simulink subsystem "Radar"  (R2024b)
settings: Solver=VariableStepAuto  StartTime=0.0  StopTime=10.0  RelTol=1e-3
undefined symbols (not defined in the file or in its folder): rel_dist, rel_vel
libraries: drivinglib x1, sim3dcameralib x1, sim3dprobsensorlib x1
settings Model: Creator=Tong  LastModifiedBy=Tong

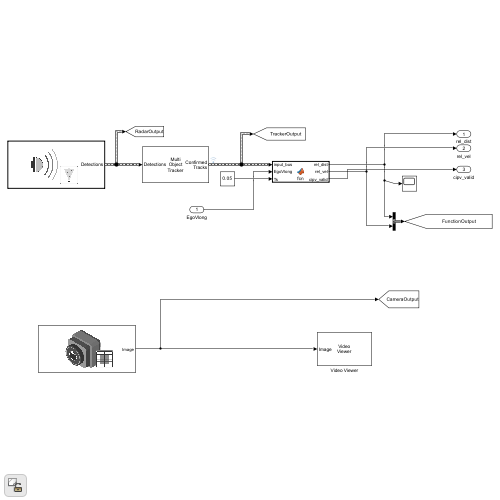
[thumbnail: Simulink's stored preview of the top-level diagram]
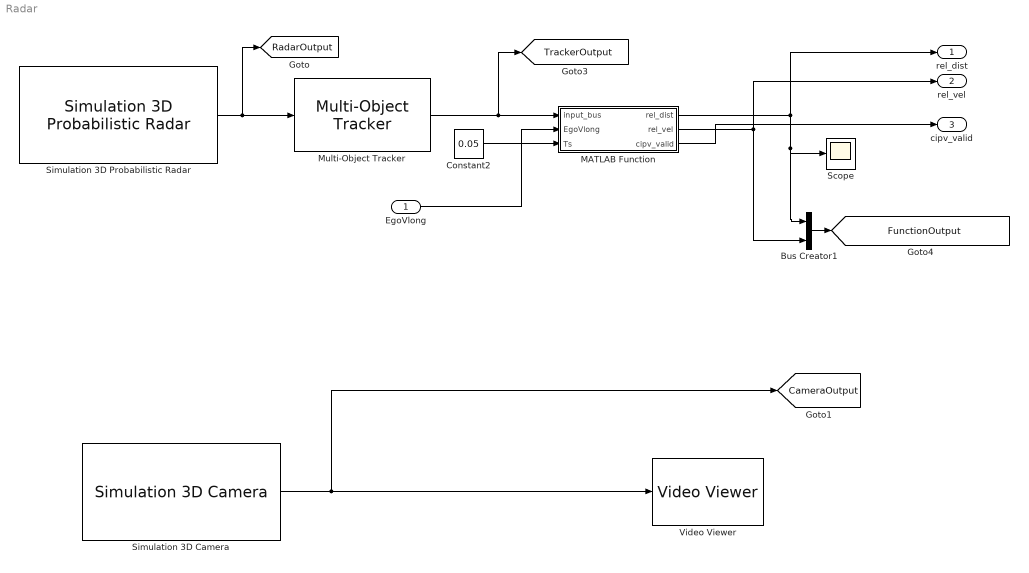
== system Radar ==
  EgoVlong : Inport
  Bus Creator1 : BusCreator  Inputs=rel_dist,rel_vel
  Constant2 : Constant  Value=0.05
  MATLAB Function : MATLAB Function  TreatAsAtomicUnit=on
  Multi-Object Tracker : drivinglib/Multi-Object Tracker  TrackerIndex=uint32( 0 )  FilterInitializationFcn=initcvekf  AssignmentThreshold=40  ConfirmationThreshold=[ 2, 3 ]  DeletionThreshold=[ 4, 5 ]  MaxNumTracks=50  MaxNumSensors=1  OOSMHandling=Terminate  StateParametersSimulink=struct  HasStateParametersInput=off  TimeInputSource=Auto  HasCostMatrixInput=off  HasDetectableTrackIDsInput=off  BusNameSource=Auto  BusName=BusMultiObjectTracker  TentativeTracksOutputPort=off  AllTracksOutputPort=off  SimulateUsing=Interpreted execution
  Scope : Scope
  Simulation 3D Camera : sim3dcameralib/Simulation 3D Camera  Priority=1  sensorTag=Sim3dSensor  sensorId=1  sensorName=Sim3dSensor  vehTagList={'Scene Origin'}  vehTag=Scene Origin  mountLoc=Hood center  offsetFlag=on  tmountOffset=[0, 0, 0]  extTmount=off  rmountOffset=[0, 0, 0]  extRmount=off  FocalLength=[1109, 1109]  OpticalCenter=[640, 360]  ImageSize=[720, 1280]  RadialDistortion=[0, 0]  TangentialDistortion=[0, 0]  SensorSkew=0  DepthOutportEnabled=off  SemanticOutportEnabled=off  TransformOutportEnabled=off  SampleTime=-1  mountPoint=[2.4735 0 0.44]  mountOrientation=[0 0 0]  aMode=3  ID=1
      settings: LibrarySourceBlock=drivingsim3d/Simulation 3D Camera
  Simulation 3D Probabilistic Radar : sim3dprobsensorlib/Simulation 3D Probabilistic Radar  Priority=1  sensorTag=Sim3dSensor  sensorId=2  sensorName=Sim3dSensor  vehTagList={'Scene Origin'}  vehTag=Scene Origin  mountLoc=Front bumper  offsetFlag=on  tmountOffset=[0.5, 0, 0.6]  rmountOffset=[0, 2, 0]  AzimuthResolution=4  ElevationResolution=5  RangeResolution=2.5  RangeRateResolution=0.5  AzimuthBiasFraction=0.1  ElevationBiasFraction=0.1  RangeBiasFraction=0.05  RangeRateBiasFraction=0.05  FieldOfView=[ 20, 6 ]  DetectionRange=[ 0.5, 150 ]  RangeRateLimits=[ -100, 100 ]  DetectionProbability=0.95  FalseAlarmRate=1e-7  ReferenceRange=200  ReferenceRCS=-15  HasElevation=on  HasRangeRate=on  HasNoise=off  HasFalseAlarms=off  InitialSeedSource=Repeatable  InitialSeed=0  MaxNumDetections=50  DetectionCoordinates=Ego Cartesian  SpecifyOutputBusName=off  BusName=BusSimulation3DRadarTruthSensor  SampleTime=0.05  mountPoint=[2.9735 0 1.04]  mountOrientation=[0 -2 0]  aMode=3  ID=2
      settings: LibrarySourceBlock=drivingsim3d/Simulation 3D Probabilistic Radar
  Video Viewer : VideoViewer  FigPos=[-8.33333333333333 995.333333333333 850.666666666667 403.333333333333]
  rel_dist : Outport
  rel_vel : Outport  Port=2
  cipv_valid : Outport  Port=3
  tag scope: CameraOutput=global, FunctionOutput=global, RadarOutput=global, TrackerOutput=global
  wires:
  Constant2/1 -> MATLAB Function/3(Ts)
  Bus Creator1/1 -> [FunctionOutput]
  Simulation 3D Probabilistic Radar/1 -> [RadarOutput], Multi-Object Tracker/1
  EgoVlong/1 -> MATLAB Function/2(EgoVlong)
  Multi-Object Tracker/1 -> MATLAB Function/1(input_bus), [TrackerOutput]
  MATLAB Function/2(rel_vel) -> rel_vel/1, Bus Creator1/2
  MATLAB Function/1(rel_dist) -> Bus Creator1/1, Scope/1, rel_dist/1
  MATLAB Function/3(cipv_valid) -> cipv_valid/1
  Simulation 3D Camera/1 -> Video Viewer/1, [CameraOutput]

== matlab function Radar/MATLAB Function ==
  settings: updateMethod=DISCRETE
  data: input_bus input; rel_dist output; rel_vel output; EgoVlong input; cipv_valid output; Ts input
function [rel_dist, rel_vel, cipv_valid] = fcn(input_bus, EgoVlong, Ts)
%#codegen
coder.extrinsic('fprintf');

% ===== 参数（按需调）=====
dNoTarget = 200;          % 无目标输出距离
dMaxOut   = 150;          % 认为有效输出的最大距离
max_coast_time = 0.5;     % 允许丢目标后靠预测维持的时间(s)
max_coast = int32(round(max_coast_time / Ts));

% KF 过程噪声（匀加速模型）
sigma_a = 2.0;            % m/s^2
% =========================

% ======= 持久变量 =======
persistent X_est P frame_count lost_count last_cipv_id inited
if isempty(inited)
    frame_count  = 0;
    lost_count   = int32(max_coast+1);  % 一开始当作无目标
    last_cipv_id = uint32(0);
    X_est = [dNoTarget; 0];
    P     = [100 0; 0 100];
    inited = true;
end

frame_count = frame_count + 1;

num_tracks  = double(input_bus.NumTracks);
tracks      = input_bus.Tracks;

% ======= 1) KF 预测 =======
dt = Ts;
A = [1 dt; 0 1];
Q = [0.25*dt^4  0.5*dt^3;
     0.5*dt^3   dt^2    ] * (sigma_a^2);

X_pred = A * X_est;
P_pred = A * P * A' + Q;

% ======= 2) 选 CIPV =======
best_idx  = -1;
best_dist = inf;

for i = 1:num_tracks
    if ~tracks(i).IsConfirmed
        continue;
    end

    st = tracks(i).State;
    x_rel  = st(1);    % 前向距离 (m)
    vx_rel = st(2);    % 相对速度 (m/s) = v_lead_long - v_ego_long（通常是这个定义）
    y_rel  = st(3);    % 横向偏移 (m)

    % ROI：纵向范围
    if x_rel < 0.5 || x_rel > dMaxOut
        continue;
    end

    % 横向走廊（可保持你原来的自适应）
    if x_rel < 10
        lane_half_width = 3.5;
    elseif x_rel < 50
        lane_half_width = 2.5;
    else
        lane_half_width = 2.0;
    end
    if abs(y_rel) > lane_half_width
        continue;
    end

    % 静态杂波过滤（注意：EgoVlong 必须是“前向速度”，不能用世界X速度）
    obj_abs_v = vx_rel + EgoVlong;
    is_ego_fast  = (EgoVlong > 5.0);
    is_obj_static = (abs(obj_abs_v) < 1.0);

    if is_ego_fast && is_obj_static && (x_rel < 25)
        % 轨迹保持：如果是上一帧CIPV尽量别滤掉
        if tracks(i).TrackID ~= last_cipv_id
            continue;
        end
        if tracks(i).Age < 10
            continue;
        end
    end

    % 最近优先
    if x_rel < best_dist
        best_dist = x_rel;
        best_idx  = i;
    end
end

% ======= 3) KF 更新 / Coast =======
if best_idx ~= -1
    st = tracks(best_idx).State;
    Z_meas = [st(1); st(2)];

    last_cipv_id = tracks(best_idx).TrackID;

    % 测量噪声（按距离自适应）
    if st(1) < 20
        R = [0.5 0; 0 5];
    elseif st(1) < 80
        R = [1.0 0; 0 20];
    else
        R = [2.0 0; 0 50];
    end

    H = eye(2);
    innovation = Z_meas - H * X_pred;
    S = H * P_pred * H' + R;
    maha = innovation' / S * innovation;

    if maha < 16
        K = P_pred * H' / S;
        X_est = X_pred + K * innovation;
        P = (eye(2) - K * H) * P_pred;
        lost_count = int32(0);
    else
        % 门控拒绝 -> 用预测（仍算“短时有效”，由 lost_count 控制）
        X_est = X_pred;
        P = P_pred;
        lost_count = min(lost_count + 1, int32(max_coast+1));

        fprintf('[GATE REJECT] Frame %d | maha=%.2f | meas=[%.1f %.1f] pred=[%.1f %.1f]\n', ...
            frame_count, maha, Z_meas(1), Z_meas(2), X_pred(1), X_pred(2));
    end

else
    % 真丢目标：coast 一段时间
    if lost_count <= max_coast
        X_est = X_pred;
        P = P_pred;
        lost_count = lost_count + 1;
    else
        X_est = [dNoTarget; 0];
        P = [100 0; 0 100];
        last_cipv_id = uint32(0);
        lost_count = int32(max_coast+1);
    end
end

% ======= 4) 输出 =======
rel_dist = max(X_est(1), 0);   % 不允许负
rel_vel  = X_est(2);

% 关键：coast 期间依然认为目标有效（否则ACC会抖）
cipv_valid = double( (rel_dist < dMaxOut) && (lost_count <= max_coast) );

% 可选调试
if mod(frame_count, 20) == 0
    fprintf('Frame %d | best=%d | lost=%d | dist=%.2f | vrel=%.2f | valid=%d\n', ...
        frame_count, (best_idx~=-1), lost_count, rel_dist, rel_vel, cipv_valid);
end

end



% function [rel_dist, rel_vel, cipv_valid] = fcn(input_bus, EgoVx)
% %#codegen
%     coder.extrinsic('fprintf');
% 
%     dt = 0.01; 
% 
%     % ======= 持久变量 =======
%     persistent X_est P frame_count hold_count last_cipv_id
%     if isempty(frame_count)
%         frame_count  = 0;
%         hold_count   = 0;
%         last_cipv_id = uint32(0);
%         X_est = [200; 0];
%         P     = [100 0; 0 100];
%     end
% 
%     frame_count = frame_count + 1;
%     num_tracks  = double(input_bus.NumTracks);
%     tracks      = input_bus.Tracks;
% 
%     % ======= 1. 卡尔曼预测 =======
%     A = [1 dt; 0 1];
%     Q = [0.25*dt^4  0.5*dt^3;    % 基于匀加速模型的过程噪声
%          0.5*dt^3   dt^2    ] * 4.0;  % σ_a^2 = 4 m/s^2 (加速度标准差2)
% 
%     X_pred = A * X_est;
%     P_pred = A * P * A' + Q;
% 
%     % ======= 2. CIPV 选择（修复近距离丢失）=======
%     best_idx  = -1;
%     best_dist = inf;
% 
%     for i = 1:num_tracks
%         st = tracks(i).State;
%         x_rel  = st(1);    % 纵向距离
%         vx_rel = st(2);    % 纵向相对速度
%         y_rel  = st(3);    % 横向偏移
% 
%         % --- 基本有效性检查 ---
%         if ~tracks(i).IsConfirmed
%             continue;
%         end
% 
%         % --- ROI: 纵向 (2m ~ 150m) ---
%         % 近距离下限从0改为2m，防止自车保险杠反射
%         if x_rel < 2 || x_rel > 150
%             continue;
%         end
% 
%         % --- ROI: 横向自适应走廊 ---
%         % 近距离放宽（雷达角度误差放大），远距离收窄
%         if x_rel < 10
%             lane_half_width = 3.5;    % 近距离：±3.5m
%         elseif x_rel < 50
%             lane_half_width = 2.5;    % 中距离：±2.5m
%         else
%             lane_half_width = 2.0;    % 远距离：±2.0m
%         end
% 
%         if abs(y_rel) > lane_half_width
%             continue;
%         end
% 
%         % --- 静态杂波过滤（关键修复！）---
%         obj_abs_v = vx_rel + EgoVx;
% 
%         % 方案：只在自车高速行驶时才过滤静态物体
%         % 如果自车速度很低 (<5m/s)，前车停着也是正常的，不应过滤
%         is_ego_moving_fast = (EgoVx > 5.0);
%         is_object_static   = (abs(obj_abs_v) < 1.0);
% 
%         % 只有在自车快速行驶时，才把近处的静态目标当杂波过滤
%         % 同时增加额外条件：如果该目标就是上一帧的CIPV，不过滤！（航迹保持）
%         if is_ego_moving_fast && is_object_static && (x_rel < 25)
%             % 检查是不是上一帧跟踪的同一个目标
%             if tracks(i).TrackID ~= last_cipv_id
%                 continue;  % 不是上帧目标，且是静态近处杂波，跳过
%             end
%             % 如果是上帧CIPV，再看 Age：如果这个航迹活了很久，说明不是杂波
%             if tracks(i).Age < 10
%                 continue;
%             end
%         end
% 
%         % --- 选最近目标 ---
%         if x_rel < best_dist
%             best_dist = x_rel;
%             best_idx  = i;
%         end
%     end
% 
%     % ======= 3. 卡尔曼更新 =======
%     if best_idx ~= -1
%         st = tracks(best_idx).State;
%         Z_meas = [st(1); st(2)];
% 
%         % 保存当前 CIPV 的 TrackID，下一帧用于航迹保持
%         last_cipv_id = tracks(best_idx).TrackID;
% 
%         H = [1 0; 0 1];
% 
%         % 自适应测量噪声：距离越近，雷达越准
%         if st(1) < 20
%             R = [0.5 0; 0 5];    % 近距离：非常信任雷达
%         elseif st(1) < 80
%             R = [1.0 0; 0 20];   % 中距离
%         else
%             R = [2.0 0; 0 50];   % 远距离：速度测量噪声大
%         end
% 
%         % ---- 新增：门控 (Gating) 防跳变 ----
%         innovation = Z_meas - H * X_pred;
%         S = H * P_pred * H' + R;
%         maha_dist = innovation' / S * innovation;  % 马氏距离
% 
%         if maha_dist < 16  % χ²(2自由度) 的 99.7% 门限 ≈ 11.8，放宽到16
%             % 正常更新
%             K = P_pred * H' / S;
%             X_est = X_pred + K * innovation;
%             P = (eye(2) - K * H) * P_pred;
%             hold_count = 0;
%         else
%             % 观测值跟预测差太远 → 可能是目标跳变/换目标，不信任此次观测
%             X_est = X_pred;
%             P = P_pred;
%             % 不重置 hold_count，让它慢慢涨
%             hold_count = hold_count + 1;
%             fprintf('[GATE REJECT] Frame %d | MahaDist=%.2f | Meas=[%.1f, %.1f] | Pred=[%.1f, %.1f]\n', ...
%                 frame_count, maha_dist, Z_meas(1), Z_meas(2), X_pred(1), X_pred(2));
%         end
%     else
%         % 无目标 → Coast
%         max_coast = 50;  % 0.5秒 (dt=0.01)
%         if hold_count < max_coast && X_est(1) < 180
%             X_est = X_pred;
%             P = P_pred;
%             hold_count = hold_count + 1;
%         else
%             X_est = [200; 0];
%             P = [100 0; 0 100];
%             last_cipv_id = uint32(0);
%         end
%     end
% 
%     % ======= 4. 输出约束 =======
%     % 距离不能为负
%     if X_est(1) < 0
%         X_est(1) = 0;
%     end
% 
%     rel_dist  = X_est(1);
%     rel_vel   = X_est(2);
%     cipv_valid = double(hold_count == 0 && rel_dist < 150);
% 
%     % 调试
%     if mod(frame_count, 10) == 0
%         fprintf('Frame %d | CIPV=%d | Coast=%d | Dist=%.2f | Vel=%.2f | Valid=%d\n', ...
%             frame_count, (best_idx~=-1), hold_count, rel_dist, rel_vel, cipv_valid);
%     end
% end

% function [rel_dist, rel_vel] = fcn(input_bus, EgoVx)
% %#codegen
%     coder.extrinsic('fprintf');
% 
%     % 仿真步长 (根据你的 Simulink 求解器设置，通常是 0.01 或 0.02)
%     dt = 0.01; 
% 
%     % ======= 卡尔曼滤波器状态初始化 =======
%     % X_est = [距离; 相对速度]
%     persistent X_est P frame_count hold_count
%     if isempty(frame_count)
%         frame_count = 0;
%         hold_count  = 0;
%         X_est = [200; 0];        % 初始状态：距离200m，相对速度0
%         P = [100 0; 0 100];      % 初始协方差矩阵（极其不信任初始值）
%     end
% 
%     frame_count = frame_count + 1;
%     num_tracks = double(input_bus.NumTracks);
%     tracks = input_bus.Tracks;
% 
%     % ======= 1. 卡尔曼滤波：预测阶段 (Predict) =======
%     % 状态转移矩阵 A: d(k) = d(k-1) + v(k-1)*dt, v(k) = v(k-1)
%     A = [1 dt; 0 1];
%     % 过程噪声 Q (假设加速度带来了噪声)
%     Q = [0.1 0; 0 1.0]; 
% 
%     X_pred = A * X_est;           % 预测当前帧的距离和速度
%     P_pred = A * P * A' + Q;      % 预测协方差
% 
%     % ======= 2. 遍历雷达航迹，寻找最危险目标 (CIPV) =======
%     best_idx = -1;
%     best_dist = inf;
% 
%     for i = 1:num_tracks
%         st = tracks(i).State;
%         x_rel  = st(1);
%         vx_rel = st(2);
%         y_rel  = st(3);
% 
%         % 过滤条件1: 只用 confirmed 且生存了一定时间的航迹
%         if ~tracks(i).IsConfirmed || tracks(i).Age < 3
%             continue;
%         end
% 
%         % 过滤条件2: ROI 感知走廊 (纵向 0~120m，横向拓宽至 2.5m 防止弯道丢失)
%         if x_rel <= 0 || x_rel > 120 || abs(y_rel) > 2.5
%             continue;
%         end
% 
%         % 过滤条件3: 静态杂波/地面鬼影剔除 (彻底解决掉到10m的问题!)
%         % 目标的绝对速度 = 相对速度 + 自车速度
%         obj_abs_v = vx_rel + EgoVx;
%         % 如果绝对速度接近 0 (小于 1.5m/s)，并且离得很近，大概率是地面井盖或护栏
%         if (x_rel < 30) && (abs(obj_abs_v) < 1.5)
%             continue;
%         end
% 
%         % 寻找距离最近的有效目标
%         if x_rel < best_dist
%             best_dist = x_rel;
%             best_idx = i;
%         end
%     end
% 
%     % ======= 3. 卡尔曼滤波：更新阶段 (Update) =======
%     if best_idx ~= -1
%         % 【情况 A：雷达成功看到了目标】
%         st = tracks(best_idx).State;
%         Z_meas = [st(1); st(2)]; % 雷达测量值 Z = [观测距离; 观测速度]
% 
%         % 测量矩阵 H 和 测量噪声 R (雷达测距准，测速极度不准，所以给速度极大的噪声方差)
%         H = [1 0; 0 1];
%         R = [2 0; 0 50]; 
% 
%         % 计算卡尔曼增益 K
%         K = P_pred * H' / (H * P_pred * H' + R);
% 
%         % 修正状态
%         X_est = X_pred + K * (Z_meas - H * X_pred);
%         P = (eye(2) - K * H) * P_pred;
% 
%         hold_count = 0; % 重置丢失计数器
%     else
%         % 【情况 B：雷达发生断闪丢失 (Coast 机制)】
%         % 容忍丢失帧数放大到 50 帧 (假设0.01s步长，即容忍 0.5 秒的纯瞎眼)
%         if hold_count < 50 && X_est(1) < 150
%             % 雷达瞎了，我们不相信观测，直接把预测值当作当前真实值！
%             % 这就是卡尔曼滤波最牛的地方：用上一秒的速度，继续往前推演距离
%             X_est = X_pred; 
%             P = P_pred;
%             hold_count = hold_count + 1;
%         else
%             % 彻底丢失前车 (超过0.5秒还没找到，或者距离太远)，复位巡航状态
%             X_est = [200; 0];
%             P = [100 0; 0 100];
%         end
%     end
% 
%     % ======= 输出平滑后的最终信号 =======
%     rel_dist = X_est(1);
%     rel_vel  = X_est(2);
% 
%     % 打印调试
%     if mod(frame_count, 10) == 0
%         fprintf('Frame %d | ValidTarget=%d | Coast=%d | OutDist=%.2f | OutVel=%.2f\n', ...
%             frame_count, (best_idx~=-1), hold_count, rel_dist, rel_vel);
%     end
% end

% function [rel_dist, rel_vel] = fcn(input_bus, EgoVx)
% %#codegen
%     coder.extrinsic('fprintf');
% 
%     rel_dist = 200;
%     rel_vel  = 0;
% 
%     persistent frame_count
%     if isempty(frame_count)
%         frame_count = 0;
%     end
%     frame_count = frame_count + 1;
% 
%     num_tracks = double(input_bus.NumTracks);
%     tracks = input_bus.Tracks;
% 
%     % 每 10 帧打印一次，避免刷屏
%     if mod(frame_count,10) == 0
%         fprintf('\n===== Frame %d | NumTracks = %d | EgoVx = %.2f =====\n', ...
%             frame_count, num_tracks, EgoVx);
% 
%         max_print = min(num_tracks, 3);
%         for i = 1:max_print
%             st = tracks(i).State;
% 
%             fprintf(['Track %d | ID=%d | Age=%.0f | Confirmed=%d | Coasted=%d | ' ...
%                      'x=%.2f | vx=%.2f | y=%.2f | vy=%.2f | SNR=%.2f\n'], ...
%                 i, ...
%                 double(tracks(i).TrackID), ...
%                 double(tracks(i).Age), ...
%                 logical(tracks(i).IsConfirmed), ...
%                 logical(tracks(i).IsCoasted), ...
%                 st(1), st(2), st(3), st(4), ...
%                 double(tracks(i).ObjectAttributes.SNR));
%         end
%     end
% 
%     % 临时逻辑：只选 confirmed 且年龄足够的最近目标
%     best_idx = -1;
%     best_dist = inf;
% 
%     for i = 1:num_tracks
%         st = tracks(i).State;
% 
%         x_rel  = st(1);
%         vx_rel = st(2);
%         y_rel  = st(3);
% 
%         if ~tracks(i).IsConfirmed
%             continue;
%         end
% 
%         if tracks(i).Age < 2
%             continue;
%         end
% 
%         if x_rel <= 0 || x_rel > 120
%             continue;
%         end
% 
%         if abs(y_rel) > 2.0
%             continue;
%         end
% 
%         if x_rel < best_dist
%             best_dist = x_rel;
%             best_idx = i;
%         end
%     end
% 
%     if best_idx ~= -1
%         st = tracks(best_idx).State;
%         rel_dist = st(1);
%         rel_vel  = st(2);
%     end
% end


% function [rel_dist, rel_vel] = fcn(input_bus, EgoVx)
% %#codegen
%     coder.extrinsic('fprintf');
% 
%     rel_dist = 200;
%     rel_vel  = 0;
% 
%     persistent frame_count last_dist last_vel hold_count
%     if isempty(frame_count)
%         frame_count = 0;
%         last_dist   = 200;
%         last_vel    = 0;
%         hold_count  = 0;
%     end
% 
%     frame_count = frame_count + 1;
%     do_print = (mod(frame_count,10) == 0);
% 
%     num_tracks = double(input_bus.NumTracks);
%     tracks = input_bus.Tracks;
% 
%     best_idx = -1;
%     best_dist = inf;
% 
%     for i = 1:num_tracks
%         st = tracks(i).State;
% 
%         x_rel  = st(1);
%         vx_rel = st(2);
%         y_rel  = st(3);
% 
%         % 1) 只用 confirmed
%         if ~tracks(i).IsConfirmed
%             continue;
%         end
% 
%         % 2) 年龄太小先不要
%         if tracks(i).Age < 3
%             continue;
%         end
% 
%         % 3) 前方范围
%         if x_rel <= 0 || x_rel > 120
%             continue;
%         end
% 
%         % 4) 横向门限
%         if abs(y_rel) > 2.0
%             continue;
%         end
% 
%         % % 5) 静止背景鬼影过滤
%         % % 如果目标绝对速度接近 0，并且在车前近距离，就认为是地面/固定物鬼影
%         % obj_abs_v = vx_rel + EgoVx;
%         % if (x_rel < 15) && (abs(y_rel) < 1.5) && (abs(obj_abs_v) < 2.0)
%         %     continue;
%         % end
%         % 
%         % % 6) 极近距离仍然直接不要
%         % if x_rel < 7.5
%         %     continue;
%         % end
% 
%         % 7) 最近目标优先
%         if x_rel < best_dist
%             best_dist = x_rel;
%             best_idx = i;
%         end
%     end
% 
%     if best_idx ~= -1
%         st = tracks(best_idx).State;
%         rel_dist = st(1);
%         rel_vel  = st(2);
%         last_dist = rel_dist;
%         last_vel  = rel_vel;
%         hold_count = 0;
%     else
%         % 短时保持
%         if hold_count < 5 && last_dist < 200
%             rel_dist = last_dist;
%             rel_vel  = last_vel;
%             hold_count = hold_count + 1;
%         else
%             rel_dist = 200;
%             rel_vel  = 0;
%             last_dist = 200;
%             last_vel  = 0;
%             hold_count = 0;
%         end
%     end
% 
%     if do_print
%         fprintf('Frame %d | NumTracks=%d | OutDist=%.2f | OutVel=%.2f\n', ...
%             frame_count, num_tracks, rel_dist, rel_vel);
%     end
% end
